simulink model "inverse_kinematics"  (Simulink 7.9)
settings: Solver=ode45  StartTime=0.0  StopTime=10.0  RelTol=1e-3
values from neighbouring files (symbols this model uses):
  initial_eta = [0,0,0,0,0,0]    [kinematic_parameters.m]
  initial_q = [0,20*d2r,-(20+25)*d2r,25*d2r,-90*d2r,0]    [kinematic_parameters.m]
  v_ee_c = [0.1,0,0,0,0.2,0]    [kinematic_parameters.m]
undefined symbols (not defined in the file or in its folder): initial_ee_pose, inner_motion_vec
libraries: simulink x3
settings Model: Creator=simena  LastModifiedBy=simena  SimulationMode=accelerator

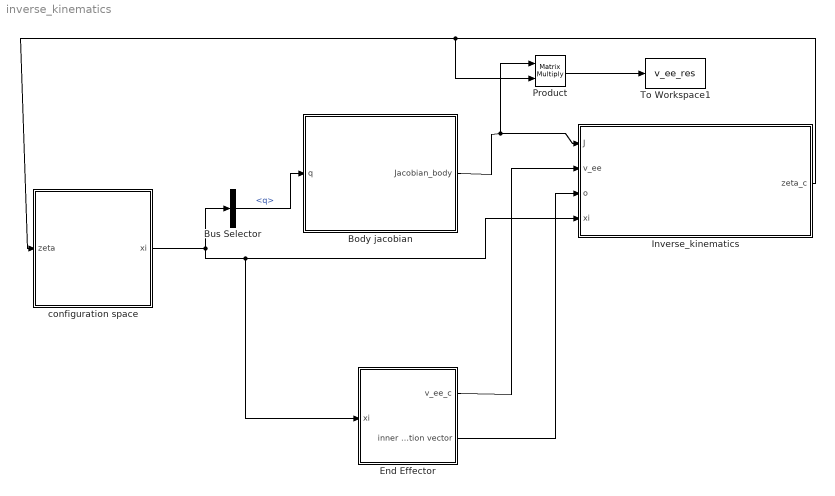
== system inverse_kinematics ==
  Body jacobian : MATLAB Function  TreatAsAtomicUnit=on
  Bus Selector : BusSelector  OutputSignals=q
  End Effector : Subsystem
  "Inverse_kinematics " : Subsystem
  Product : Product  Multiplication=Matrix(*)  RndMeth=Zero
  To Workspace1 : ToWorkspace  VariableName=v_ee_res  SampleTime=-1  SaveFormat=Structure With Time
  configuration space : Subsystem
  wires:
  configuration space/1(xi) -> Bus Selector/1, "Inverse_kinematics "/4(xi), End Effector/1(xi)
  Bus Selector/1 -> Body jacobian/1(q)  "<q>"
  "Inverse_kinematics "/1(zeta_c) -> configuration space/1(zeta), Product/2
  Body jacobian/1(Jacobian_body) -> "Inverse_kinematics "/1(J), Product/1
  End Effector/2(inner motion vector) -> "Inverse_kinematics "/3(o)
  Product/1 -> To Workspace1/1
  End Effector/1(v_ee_c) -> "Inverse_kinematics "/2(v_ee)

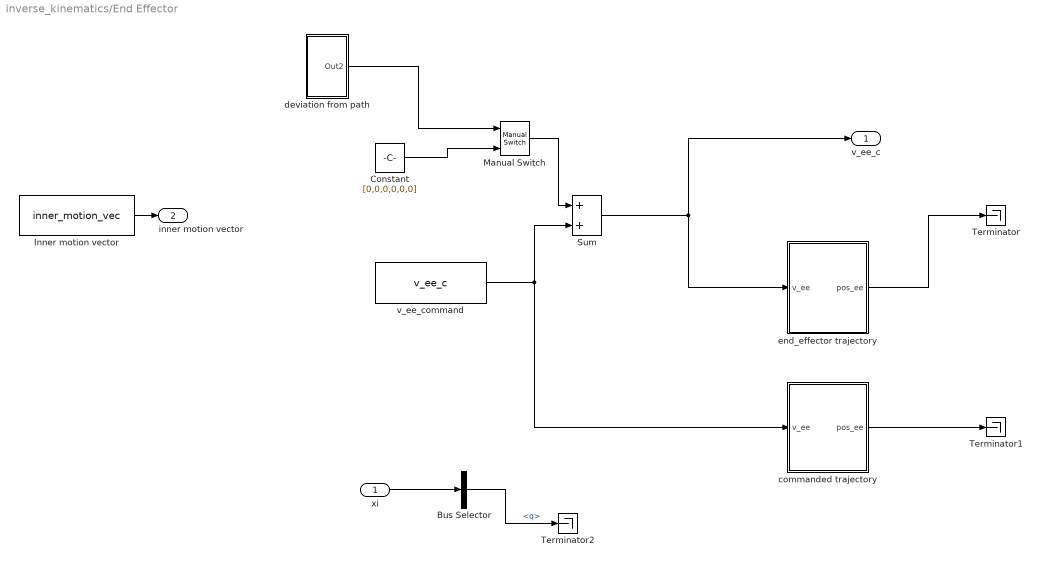
== system inverse_kinematics/End Effector ==
  xi : Inport
  Bus Selector : BusSelector  OutputSignals=q
  Constant : Constant  Value=[0,0,0,0,0,0]
  Inner motion vector : Constant  Value=inner_motion_vec
  Manual Switch : simulink/Signal Routing/Manual Switch  sw=0  action=0  varsize=off
  Sum : Sum
  Terminator : Terminator
  Terminator1 : Terminator
  Terminator2 : Terminator
  commanded trajectory : Subsystem
  deviation from path : Subsystem
  end_effector trajectory : Subsystem
  v_ee_command : Constant  Value=v_ee_c
  v_ee_c : Outport
  inner motion vector : Outport  Port=2
  wires:
  Inner motion vector/1 -> inner motion vector/1
  v_ee_command/1 -> Sum/2, commanded trajectory/1(v_ee)
  Sum/1 -> end_effector trajectory/1(v_ee), v_ee_c/1
  end_effector trajectory/1(pos_ee) -> Terminator/1
  commanded trajectory/1(pos_ee) -> Terminator1/1
  Manual Switch/1 -> Sum/1
  deviation from path/1(Out2) -> Manual Switch/1
  Constant/1 -> Manual Switch/2
  xi/1 -> Bus Selector/1
  Bus Selector/1 -> Terminator2/1  "<q>"

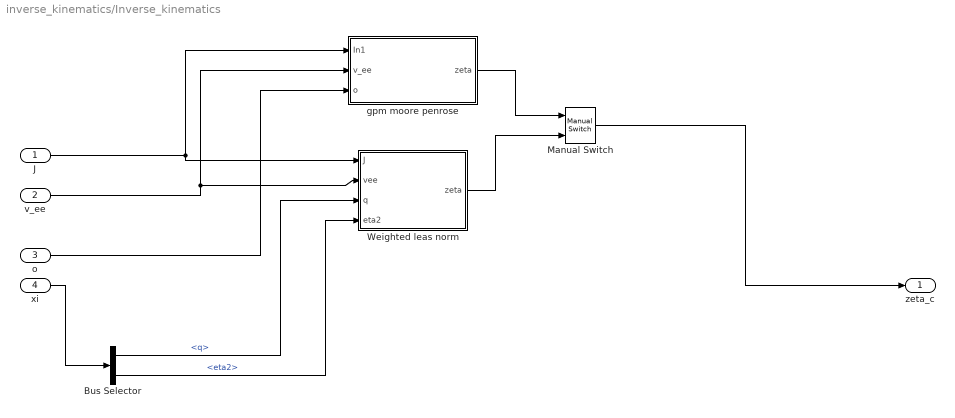
== system inverse_kinematics/Inverse_kinematics  ==
  J : Inport
  v_ee : Inport  Port=2
  o : Inport  Port=3
  xi : Inport  Port=4
  Bus Selector : BusSelector  OutputSignals=q,eta2
  Manual Switch : simulink/Signal Routing/Manual Switch  sw=0  action=0  varsize=off
  Weighted leas norm : MATLAB Function  TreatAsAtomicUnit=on
  gpm moore penrose : Subsystem
  zeta_c : Outport
  wires:
  J/1 -> gpm moore penrose/1(In1), Weighted leas norm/1(J)
  v_ee/1 -> gpm moore penrose/2(v_ee), Weighted leas norm/2(vee)
  o/1 -> gpm moore penrose/3(o)
  gpm moore penrose/1(zeta) -> Manual Switch/1
  Weighted leas norm/1(zeta) -> Manual Switch/2
  Manual Switch/1 -> zeta_c/1
  xi/1 -> Bus Selector/1
  Bus Selector/1 -> Weighted leas norm/3(q)  "<q>"
  Bus Selector/2 -> Weighted leas norm/4(eta2)  "<eta2>"

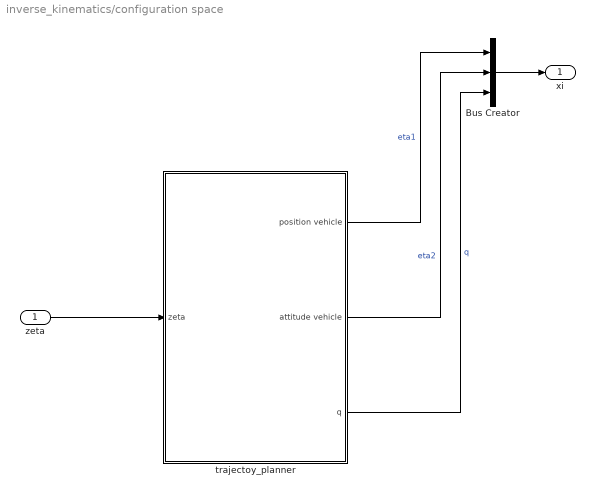
== system inverse_kinematics/configuration space ==
  zeta : Inport
  Bus Creator : BusCreator  Inputs=3
  trajectoy_planner : Subsystem
  xi : Outport
  wires:
  trajectoy_planner/1(position vehicle) -> Bus Creator/1  "eta1"
  trajectoy_planner/2(attitude vehicle) -> Bus Creator/2  "eta2"
  trajectoy_planner/3(q) -> Bus Creator/3  "q"
  Bus Creator/1 -> xi/1
  zeta/1 -> trajectoy_planner/1(zeta)

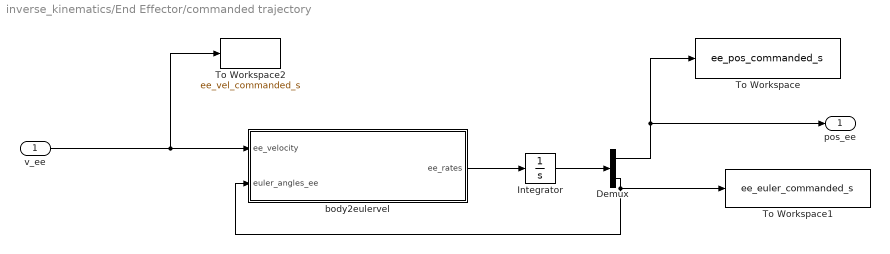
== system inverse_kinematics/End Effector/commanded trajectory ==
  v_ee : Inport
  Demux : Demux  Outputs=2
  Integrator : Integrator  InitialCondition=initial_ee_pose
  To Workspace : ToWorkspace  VariableName=ee_pos_commanded_s  SampleTime=-1  SaveFormat=Structure With Time
  To Workspace1 : ToWorkspace  VariableName=ee_euler_commanded_s  SampleTime=-1  SaveFormat=Structure With Time
  To Workspace2 : ToWorkspace  VariableName=ee_vel_commanded_s  SampleTime=-1  SaveFormat=Structure With Time
  body2eulervel : MATLAB Function  TreatAsAtomicUnit=on
  pos_ee : Outport
  wires:
  v_ee/1 -> body2eulervel/1(ee_velocity), To Workspace2/1
  body2eulervel/1(ee_rates) -> Integrator/1
  Integrator/1 -> Demux/1
  Demux/1 -> To Workspace/1, pos_ee/1
  Demux/2 -> body2eulervel/2(euler_angles_ee), To Workspace1/1

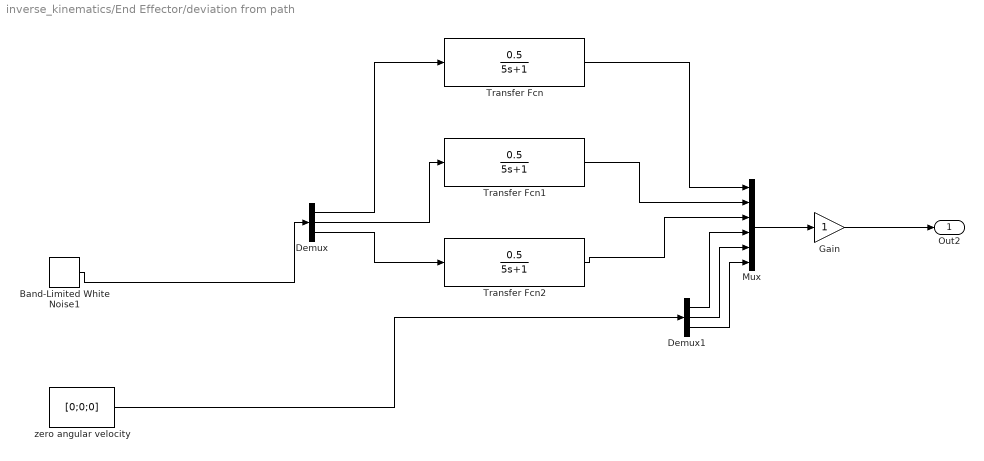
== system inverse_kinematics/End Effector/deviation from path ==
  Band-Limited White Noise1 : simulink/Sources/Band-Limited White Noise  Cov=[0.1;0.1;0.05]  Ts=0.001  seed=[23341]
  Demux : Demux  Outputs=3
  Demux1 : Demux  Outputs=3
  Gain : Gain
  Mux : Mux  Inputs=6
  Transfer Fcn : TransferFcn  Numerator=[0.5]  Denominator=[5, 1]
  Transfer Fcn1 : TransferFcn  Numerator=[0.5]  Denominator=[5, 1]
  Transfer Fcn2 : TransferFcn  Numerator=[0.5]  Denominator=[5, 1]
  zero angular velocity : Constant  Value=[0;0;0]
  Out2 : Outport
  wires:
  Band-Limited White Noise1/1 -> Demux/1
  Mux/1 -> Gain/1
  Demux/1 -> Transfer Fcn/1
  Demux/2 -> Transfer Fcn1/1
  Transfer Fcn/1 -> Mux/1
  Demux1/1 -> Mux/4
  Demux1/2 -> Mux/5
  Demux1/3 -> Mux/6
  zero angular velocity/1 -> Demux1/1
  Gain/1 -> Out2/1
  Transfer Fcn2/1 -> Mux/3
  Transfer Fcn1/1 -> Mux/2
  Demux/3 -> Transfer Fcn2/1

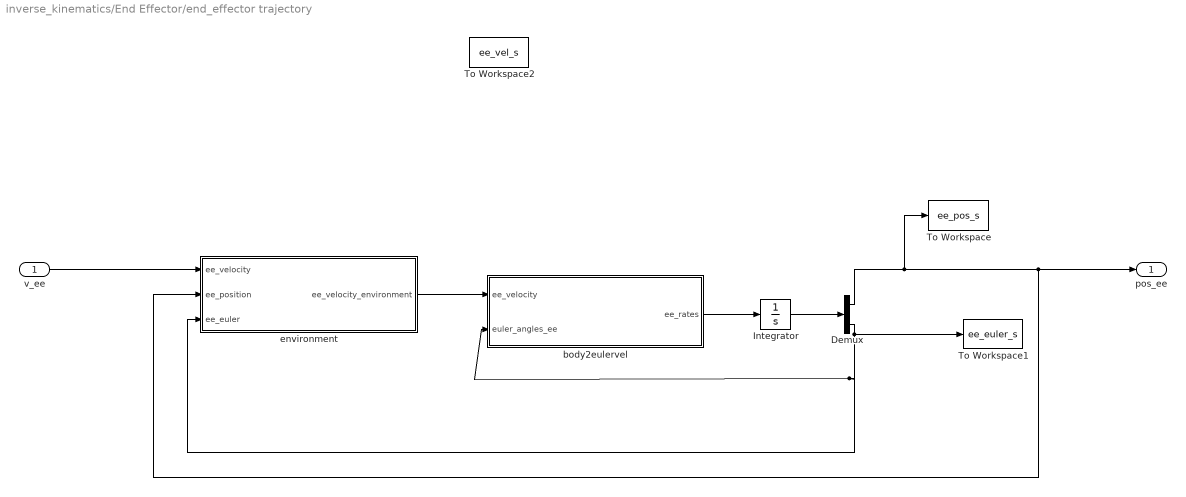
== system inverse_kinematics/End Effector/end_effector trajectory ==
  v_ee : Inport
  Demux : Demux  Outputs=2
  Integrator : Integrator  InitialCondition=initial_ee_pose
  To Workspace : ToWorkspace  VariableName=ee_pos_s  SampleTime=-1  SaveFormat=Structure With Time
  To Workspace1 : ToWorkspace  VariableName=ee_euler_s  SampleTime=-1  SaveFormat=Structure With Time
  To Workspace2 : ToWorkspace  VariableName=ee_vel_s  SampleTime=-1  SaveFormat=Structure With Time
  body2eulervel : MATLAB Function  TreatAsAtomicUnit=on
  environment : MATLAB Function  TreatAsAtomicUnit=on
  pos_ee : Outport
  wires:
  body2eulervel/1(ee_rates) -> Integrator/1
  Integrator/1 -> Demux/1
  Demux/1 -> To Workspace/1, pos_ee/1, environment/2(ee_position)
  Demux/2 -> To Workspace1/1, body2eulervel/2(euler_angles_ee), environment/3(ee_euler)
  v_ee/1 -> environment/1(ee_velocity)
  environment/1(ee_velocity_environment) -> body2eulervel/1(ee_velocity)

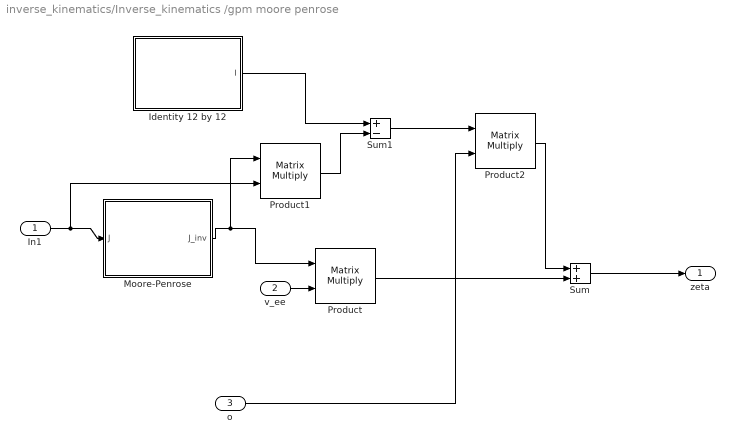
== system inverse_kinematics/Inverse_kinematics /gpm moore penrose ==
  In1 : Inport
  v_ee : Inport  Port=2
  o : Inport  Port=3
  Identity 12 by 12 : MATLAB Function  TreatAsAtomicUnit=on
  Moore-Penrose : MATLAB Function  TreatAsAtomicUnit=on
  Product : Product  Multiplication=Matrix(*)  RndMeth=Zero
  Product1 : Product  Multiplication=Matrix(*)  RndMeth=Zero
  Product2 : Product  Multiplication=Matrix(*)  RndMeth=Zero
  Sum : Sum
  Sum1 : Sum  Inputs=+-
  zeta : Outport
  wires:
  In1/1 -> Product1/2, Moore-Penrose/1(J)
  Moore-Penrose/1(J_inv) -> Product/1, Product1/1
  Product/1 -> Sum/2
  Identity 12 by 12/1(I) -> Sum1/1
  Product1/1 -> Sum1/2
  Sum1/1 -> Product2/1
  Product2/1 -> Sum/1
  v_ee/1 -> Product/2
  Sum/1 -> zeta/1
  o/1 -> Product2/2

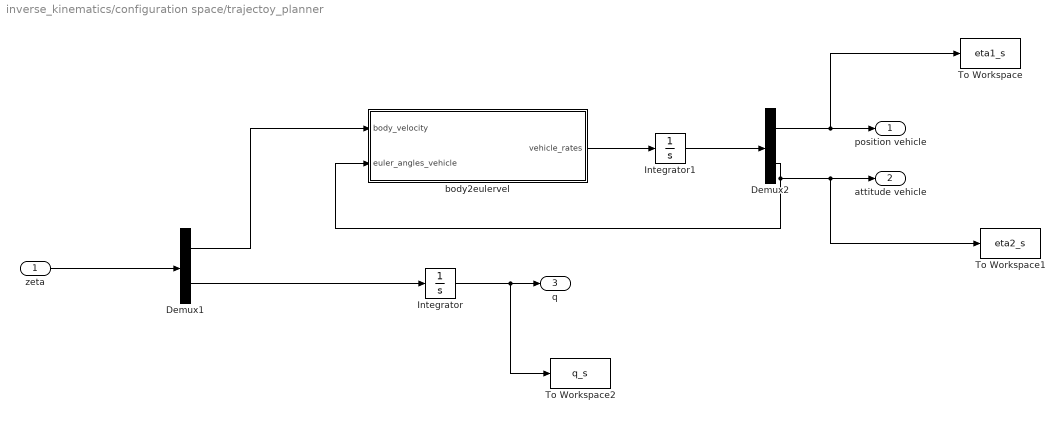
== system inverse_kinematics/configuration space/trajectoy_planner ==
  zeta : Inport
  Demux1 : Demux  Outputs=2
  Demux2 : Demux  Outputs=2
  Integrator : Integrator  InitialCondition=initial_q
  Integrator1 : Integrator  InitialCondition=initial_eta
  To Workspace : ToWorkspace  VariableName=eta1_s  SampleTime=-1  SaveFormat=Structure With Time
  To Workspace1 : ToWorkspace  VariableName=eta2_s  SampleTime=-1  SaveFormat=Structure With Time
  To Workspace2 : ToWorkspace  VariableName=q_s  SampleTime=-1  SaveFormat=Structure With Time
  body2eulervel : MATLAB Function  TreatAsAtomicUnit=on
  position vehicle : Outport
  attitude vehicle : Outport  Port=2
  q : Outport  Port=3
  wires:
  zeta/1 -> Demux1/1
  Demux1/2 -> Integrator/1
  Demux1/1 -> body2eulervel/1(body_velocity)
  Integrator/1 -> q/1, To Workspace2/1
  body2eulervel/1(vehicle_rates) -> Integrator1/1
  Integrator1/1 -> Demux2/1
  Demux2/2 -> body2eulervel/2(euler_angles_vehicle), attitude vehicle/1, To Workspace1/1
  Demux2/1 -> position vehicle/1, To Workspace/1

== matlab function Inverse_kinematics /gpm moore penrose/Identity 12 by 12 ==
  data: I output double
function I = Identity_mat()
    %#codegen
    I=eye(12);
end

== matlab function Body jacobian ==
  data: q input double; Jacobian_body output double
function Jacobian_body = fcn(q)
    %#codegen
    Jacobian_body=zeros(6,12);
    coder.extrinsic('body_jacobian');
    newq=zeros(1,6);
    newq=q;
    Jacobian_body=body_jacobian(newq);
end

== matlab function configuration space/trajectoy_planner/body2eulervel ==
  data: body_velocity input double; vehicle_rates output double; euler_angles_vehicle input double
function vehicle_rates = fcn(body_velocity, euler_angles_vehicle)                       
    %#codegen
    coder.extrinsic('analytical_jacobian');
    J=analytical_jacobian(euler_angles_vehicle);

    vehicle_rates = zeros(6,1);
    vehicle_rates=J*body_velocity;
end

== matlab function Inverse_kinematics /gpm moore penrose/Moore-Penrose ==
  data: J input double; J_inv output double
function J_inv = moore_penrose(J)
    %#codegen
    coder.extrinsic('mp_inv');
    
    J_inv=zeros(12,6);
    J_inv = mp_inv(J);
        
end

== matlab function End Effector/end_effector trajectory/body2eulervel ==
  data: ee_velocity input double; ee_rates output double; euler_angles_ee input double
function ee_rates = fcn(ee_velocity, euler_angles_ee)                       
    %#codegen
    coder.extrinsic('analytical_jacobian');
    J=analytical_jacobian(euler_angles_ee);

    ee_rates = zeros(6,1);
    ee_rates=J*ee_velocity;
end

== matlab function Inverse_kinematics /Weighted leas norm ==
  data: J input double; zeta output double; vee input double; q input double; eta2 input double
function zeta = wln(J,vee,q, eta2)
%#codegen
    coder.extrinsic('wln_m');
    J_inv=zeros(12,6);
    J_inv=wln_m(J,q,eta2);    
    
    zeta = J_inv(1:12,1:6)*vee;
end

== matlab function End Effector/commanded trajectory/body2eulervel ==
  data: ee_velocity input double; ee_rates output double; euler_angles_ee input double
function ee_rates = fcn(ee_velocity, euler_angles_ee)                       
    %#codegen
    coder.extrinsic('analytical_jacobian');
    J=analytical_jacobian(euler_angles_ee);

    ee_rates = zeros(6,1);
    ee_rates=J*ee_velocity;
end

== matlab function End Effector/end_effector trajectory/environment ==
  data: ee_velocity input double; ee_position input double; ee_velocity_environment output double; ee_euler input double
function ee_velocity_environment = velocity(ee_velocity,ee_position, ee_euler)                     
   %#codegen
   coder.extrinsic('Rzyx');
   R=Rzyx(ee_euler(1), ee_euler(2), ee_euler(3));
   ee_v_i = Rzyx * ee_velocity;
   
   
   % check for obstacle
    if ee_position(1) < 5
        % do nothing
    elseif ee_position(1) > 5
        ee_v_i(1)=0;
    elseif
                
    end
   
   
   
   
   
   ee_velocity_environment=ones(6,1);
   
   
end
